simulink model "Projekt_simulink_v2"  (R2024b)
settings: Solver=VariableStepAuto  StartTime=0.0  StopTime=150  RelTol=1e-8
values from neighbouring files (symbols this model uses):
  A = zeros(12)    [pokus_simulink.m]
  B = zeros(12, 4)    [pokus_simulink.m]
  C = eye(12)    [pokus_simulink.m]
  D = zeros(12, 4)    [pokus_simulink.m]
  g = 9.81    [pokus_simulink.m]
  Mass = 1.3    [pokus_simulink.m]
libraries: slpidlib x3
settings Model: Creator=lucie  LastModifiedBy=lucie

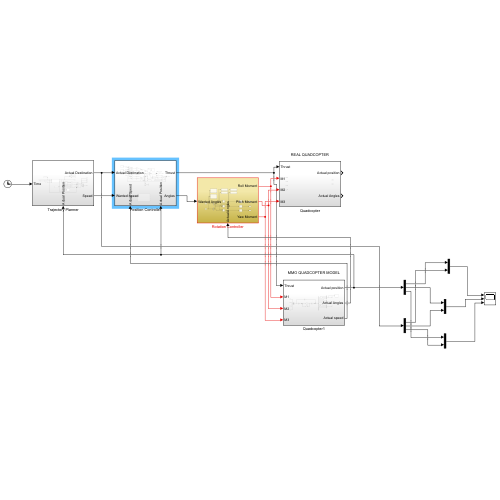
[thumbnail: Simulink's stored preview of the top-level diagram]
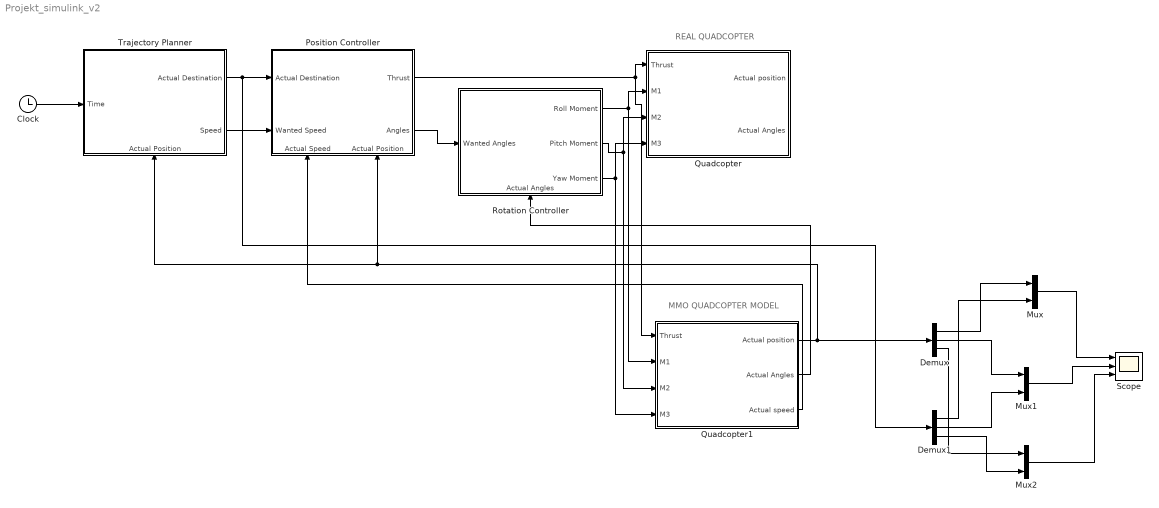
== system Projekt_simulink_v2 ==
  note: REAL QUADCOPTER
  note: MMO QUADCOPTER MODEL
  Clock : Clock
  Demux : Demux  Outputs=3
  Demux1 : Demux  Outputs=3
  Mux : Mux  Inputs=2
  Mux1 : Mux  Inputs=2
  Mux2 : Mux  Inputs=2
  Position Controller : Subsystem
      settings: PortSchema="{\"entries\":[{\"content\":{\"sides\":[{\"content\":{\"connectorIds\":[\"In1\",\"In2\"]},\"type\":\"ConnectorPlacement.EquallySpacedRectSide\",\"uuid\":\"80f29ff0-56da-481e-95f1-a9d4517a9ed9\"},{\"content\":{\"connectorIds\":[\"Out1\",\"Out2\"],\"side\":\"RIGHT\"},\"type\":\"ConnectorPlacement.EquallySpacedRectSide\",\"uuid\":\"630d0718-5a0f-420d-89e4-ff766e1306d8\"},{\"content\":{\"side\":\"TOP\"},\"type\":\"ConnectorPlacement.EquallySpacedRectSide\",\"uuid\":\"1f5a52b9-8732-4ff3-b402-4000d2af11bc\"},{\"content\":{\"connectorIds\":[\"In3\",\"In4\"],\"side\":\"BOTTOM\"},\"type\":\"ConnectorPlacement.EquallySpacedRectSide\",\"uuid\":\"db5f8e2a-d0de-4587-b83f-8eeb0fa2830b\"}]},\"type\":\"ConnectorPlacement.EquallySpacedConnector\",\"uuid\":\"97645df6-1a74-4cc0-aee4-69f235aa0ffb\"}],\"packageUris\":[\"http://schema.mathworks.com/mf0/Connector/R2020b\"],\"version\":\"1.0\"}"
  Quadcopter : Subsystem
  Quadcopter1 : Subsystem
  Rotation Controller : Subsystem
      settings: PortSchema="{\"entries\":[{\"content\":{\"sides\":[{\"content\":{\"connectorIds\":[\"In1\"]},\"type\":\"ConnectorPlacement.EquallySpacedRectSide\",\"uuid\":\"80f29ff0-56da-481e-95f1-a9d4517a9ed9\"},{\"content\":{\"connectorIds\":[\"Out1\",\"Out2\",\"Out3\"],\"side\":\"RIGHT\"},\"type\":\"ConnectorPlacement.EquallySpacedRectSide\",\"uuid\":\"630d0718-5a0f-420d-89e4-ff766e1306d8\"},{\"content\":{\"side\":\"TOP\"},\"type\":\"ConnectorPlacement.EquallySpacedRectSide\",\"uuid\":\"1f5a52b9-8732-4ff3-b402-4000d2af11bc\"},{\"content\":{\"connectorIds\":[\"In2\"],\"side\":\"BOTTOM\"},\"type\":\"ConnectorPlacement.EquallySpacedRectSide\",\"uuid\":\"db5f8e2a-d0de-4587-b83f-8eeb0fa2830b\"}]},\"type\":\"ConnectorPlacement.EquallySpacedConnector\",\"uuid\":\"97645df6-1a74-4cc0-aee4-69f235aa0ffb\"}],\"packageUris\":[\"http://schema.mathworks.com/mf0/Connector/R2020b\"],\"version\":\"1.0\"}"
  Scope : Scope  NumInputPorts=3
  Trajectory Planner : Subsystem
      settings: PortSchema="{\"entries\":[{\"content\":{\"sides\":[{\"content\":{\"connectorIds\":[\"In1\"]},\"type\":\"ConnectorPlacement.EquallySpacedRectSide\",\"uuid\":\"80f29ff0-56da-481e-95f1-a9d4517a9ed9\"},{\"content\":{\"connectorIds\":[\"Out1\",\"Out2\"],\"side\":\"RIGHT\"},\"type\":\"ConnectorPlacement.EquallySpacedRectSide\",\"uuid\":\"630d0718-5a0f-420d-89e4-ff766e1306d8\"},{\"content\":{\"side\":\"TOP\"},\"type\":\"ConnectorPlacement.EquallySpacedRectSide\",\"uuid\":\"1f5a52b9-8732-4ff3-b402-4000d2af11bc\"},{\"content\":{\"connectorIds\":[\"In2\"],\"side\":\"BOTTOM\"},\"type\":\"ConnectorPlacement.EquallySpacedRectSide\",\"uuid\":\"db5f8e2a-d0de-4587-b83f-8eeb0fa2830b\"}]},\"type\":\"ConnectorPlacement.EquallySpacedConnector\",\"uuid\":\"97645df6-1a74-4cc0-aee4-69f235aa0ffb\"}],\"packageUris\":[\"http://schema.mathworks.com/mf0/Connector/R2020b\"],\"version\":\"1.0\"}"
  wires:
  Trajectory Planner/1(Actual Destination) -> Demux1/1, Position Controller/1(Actual Destination)
  Trajectory Planner/2(Speed) -> Position Controller/2(Wanted Speed)
  Position Controller/2(Angles) -> Rotation Controller/1(Wanted Angles)
  Position Controller/1(Thrust) -> Quadcopter/1(Thrust), Quadcopter1/1(Thrust)
  Rotation Controller/1(Roll Moment) -> Quadcopter/2(M1), Quadcopter1/2(M1)
  Rotation Controller/2(Pitch Moment) -> Quadcopter1/3(M2), Quadcopter/3(M2)
  Rotation Controller/3(Yaw Moment) -> Quadcopter1/4(M3), Quadcopter/4(M3)
  Quadcopter1/2(Actual Angles) -> Rotation Controller/2(Actual Angles)
  Quadcopter1/3(Actual speed) -> Position Controller/3(Actual Speed)
  Clock/1 -> Trajectory Planner/1(Time)
  Quadcopter1/1(Actual position) -> Position Controller/4(Actual Position), Trajectory Planner/2(Actual Position), Demux/1
  Demux/1 -> Mux/1
  Demux1/1 -> Mux/2
  Demux/2 -> Mux1/1
  Demux1/2 -> Mux1/2
  Demux/3 -> Mux2/1
  Demux1/3 -> Mux2/2
  Mux/1 -> Scope/1
  Mux1/1 -> Scope/2
  Mux2/1 -> Scope/3

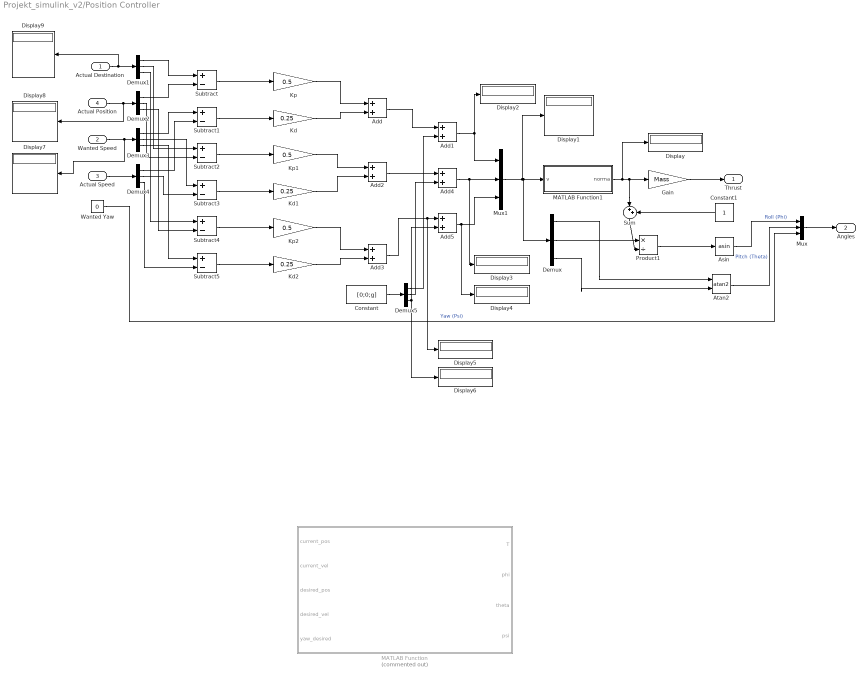
== system Projekt_simulink_v2/Position Controller ==
  Actual Destination : Inport
  Wanted Speed : Inport  Port=2
  Actual Speed : Inport  Port=3
  Actual Position : Inport  Port=4
  Add{,1..5} (6 alike) : Sum
  Asin : Trigonometry  Operator=asin
  Atan2 : Trigonometry  Operator=atan2
  Constant : Constant  Value=[0;0;g]
  Constant1 : Constant
  Demux{,1..5} (6 alike) : Demux  Outputs=3
  Display{,1..9} (10 alike) : Display
  Gain : Gain  Gain=Mass
  Kd : Gain  Gain=0.25
  Kd1 : Gain  Gain=0.25
  Kd2 : Gain  Gain=0.25
  Kp : Gain  Gain=0.5
  Kp1 : Gain  Gain=0.5
  Kp2 : Gain  Gain=0.5
  MATLAB Function : MATLAB Function  Commented=on  TreatAsAtomicUnit=on
  MATLAB Function1 : MATLAB Function  TreatAsAtomicUnit=on
  Mux : Mux  Inputs=3
  Mux1 : Mux  Inputs=3
  Product1 : Product  Inputs=*/
  Subtract{,1..5} (6 alike) : Sum  Inputs=+-
  Sum : Sum  Inputs=|++
  Wanted Yaw : Constant  Value=0
  Thrust : Outport
  Angles : Outport  Port=2
  wires:
  Mux/1 -> Angles/1
  Subtract/1 -> Kp/1
  Subtract1/1 -> Kd/1
  Kp/1 -> Add/1
  Kd/1 -> Add/2
  Gain/1 -> Thrust/1
  Actual Destination/1 -> Display9/1, Demux1/1
  Actual Position/1 -> Display8/1, Demux2/1
  Wanted Speed/1 -> Display7/1, Demux3/1
  Actual Speed/1 -> Demux4/1
  Demux1/1 -> Subtract/1
  Demux2/1 -> Subtract/2
  Demux3/1 -> Subtract1/1
  Demux4/1 -> Subtract1/2
  Kd1/1 -> Add2/2
  Subtract3/1 -> Kd1/1
  Kp1/1 -> Add2/1
  Kd2/1 -> Add3/2
  Subtract5/1 -> Kd2/1
  Kp2/1 -> Add3/1
  Subtract4/1 -> Kp2/1
  Subtract2/1 -> Kp1/1
  Demux1/2 -> Subtract2/1
  Demux2/2 -> Subtract2/2
  Demux3/2 -> Subtract3/1
  Demux4/2 -> Subtract3/2
  Demux1/3 -> Subtract4/1
  Demux2/3 -> Subtract4/2
  Demux3/3 -> Subtract5/1
  Demux4/3 -> Subtract5/2
  Constant/1 -> Demux5/1
  Add/1 -> Add1/1
  Demux5/1 -> Add1/2
  Demux5/2 -> Add4/2
  Demux5/3 -> Add5/2, Display6/1
  Add3/1 -> Display5/1, Add5/1
  Add2/1 -> Add4/1
  Add1/1 -> Display2/1, Mux1/1
  Add4/1 -> Display3/1, Mux1/2
  Add5/1 -> Display4/1, Mux1/3
  Mux1/1 -> Display1/1, Demux/1, MATLAB Function1/1(v)
  MATLAB Function1/1(norma) -> Display/1, Sum/1, Gain/1
  Demux/2 -> Product1/1
  Product1/1 -> Asin/1
  Asin/1 -> Mux/1  "Roll (Phi)"
  Demux/1 -> Atan2/1
  Demux/3 -> Atan2/2
  Atan2/1 -> Mux/2  "Pitch (Theta)"
  Wanted Yaw/1 -> Mux/3  "Yaw (Psi)"
  Constant1/1 -> Sum/2
  Sum/1 -> Product1/2

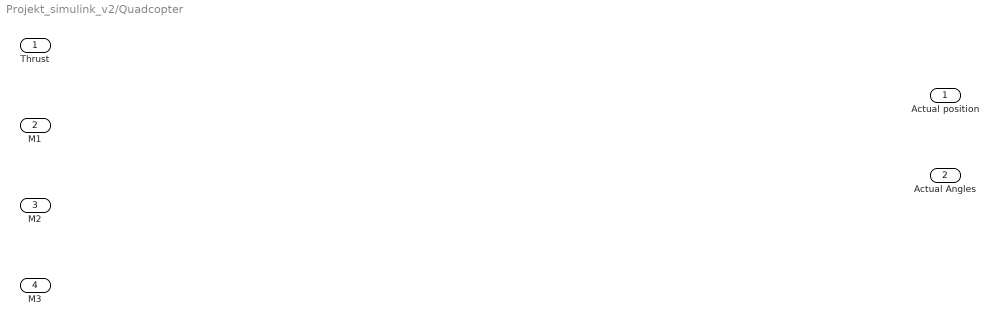
== system Projekt_simulink_v2/Quadcopter ==
  Thrust : Inport
  M1 : Inport  Port=2
  M2 : Inport  Port=3
  M3 : Inport  Port=4
  Actual position : Outport
  Actual Angles : Outport  Port=2

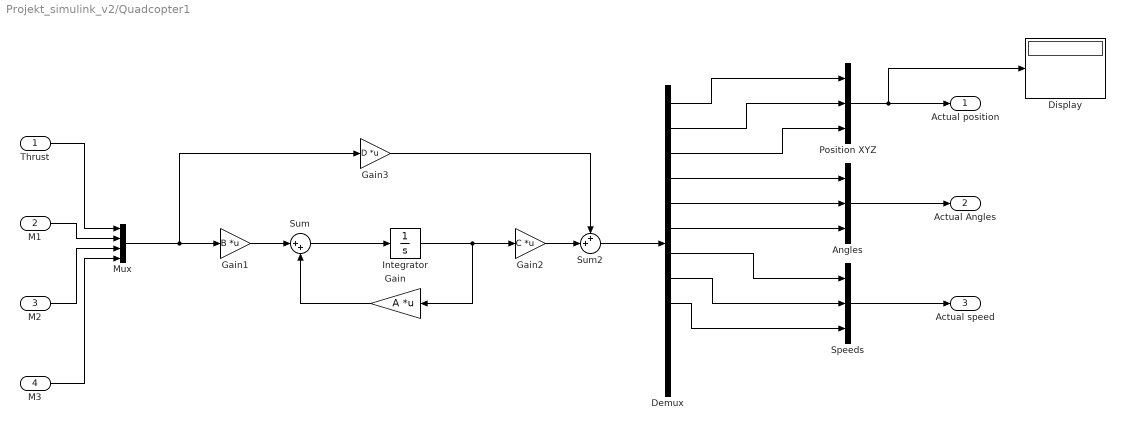
== system Projekt_simulink_v2/Quadcopter1 ==
  Thrust : Inport
  M1 : Inport  Port=2
  M2 : Inport  Port=3
  M3 : Inport  Port=4
  Angles : Mux  Inputs=3
  Demux : Demux  Outputs=12
  Display : Display
  Gain : Gain  Gain=A  Multiplication=Matrix(K*u)
  Gain1 : Gain  Gain=B  Multiplication=Matrix(K*u)
  Gain2 : Gain  Gain=C  Multiplication=Matrix(K*u)
  Gain3 : Gain  Gain=D  Multiplication=Matrix(K*u)
  Integrator : Integrator  InitialCondition=[0 0 -6 0 0 0 0 0 0 0 0 0]
  Mux : Mux
  Position XYZ : Mux  Inputs=3
  Speeds : Mux  Inputs=3
  Sum : Sum  Inputs=|++
  Sum2 : Sum  Inputs=++|
  Actual position : Outport
  Actual Angles : Outport  Port=2
  Actual speed : Outport  Port=3
  wires:
  Gain/1 -> Sum/2
  Gain1/1 -> Sum/1
  Sum/1 -> Integrator/1
  Integrator/1 -> Gain/1, Gain2/1
  Gain2/1 -> Sum2/2
  Gain3/1 -> Sum2/1
  Thrust/1 -> Mux/1
  M1/1 -> Mux/2
  M2/1 -> Mux/3
  M3/1 -> Mux/4
  Mux/1 -> Gain3/1, Gain1/1
  Sum2/1 -> Demux/1
  Demux/1 -> Position XYZ/1
  Demux/3 -> Position XYZ/3
  Demux/2 -> Position XYZ/2
  Position XYZ/1 -> Display/1, Actual position/1
  Demux/4 -> Angles/1
  Demux/5 -> Angles/2
  Demux/6 -> Angles/3
  Angles/1 -> Actual Angles/1
  Demux/7 -> Speeds/1
  Demux/8 -> Speeds/2
  Demux/9 -> Speeds/3
  Speeds/1 -> Actual speed/1

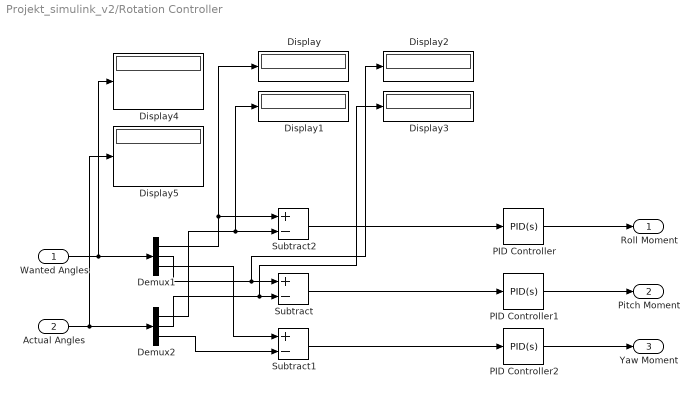
== system Projekt_simulink_v2/Rotation Controller ==
  Wanted Angles : Inport
  Actual Angles : Inport  Port=2
  Demux1 : Demux  Outputs=3
  Demux2 : Demux  Outputs=3
  Display{,1..5} (6 alike) : Display
  PID Controller : slpidlib/PID Controller  Controller=PID  Form=Parallel  TimeDomain=Continuous-time  UseExternalTs=off  SampleTime=-1  IntegratorMethod=Forward Euler  FilterMethod=Forward Euler  ControllerParametersSource=internal  P=0.5  I=0.1  UseKiTs=off  D=0.05  UseExternalDerivativeSource=off  N=100  UseFilter=on  TunerSelectOption=Transfer Function Based (PID Tuner App)  InitialConditionSource=internal  InitialConditionForIntegrator=0  InitialConditionForFilter=0  DifferentiatorICPrevScaledInput=0  ExternalReset=none  TrackingMode=off  Kt=1  LimitOutput=off  SatLimitsSource=internal  UpperSaturationLimit=inf  LowerSaturationLimit=-inf  LinearizeAsGain=on  AntiWindupMode=none  Kb=1  LimitIntegrator=off  UpperIntegratorSaturationLimit=inf  LowerIntegratorSaturationLimit=-inf  POutMin=[]  POutMax=[]  IOutMin=[]  IOutMax=[]  DOutMin=[]  DOutMax=[]  NOutMin=[]  NOutMax=[]  SumOutMin=[]  SumOutMax=[]  SaturationOutMin=[]  SaturationOutMax=[]  PParamMin=[]  PParamMax=[]  IParamMin=[]  IParamMax=[]  DParamMin=[]  DParamMax=[]  NParamMin=[]  NParamMax=[]  KbParamMin=[]  KbParamMax=[]  KtParamMin=[]  KtParamMax=[]  KbOutMin=[]  KbOutMax=[]  KtOutMin=[]  KtOutMax=[]  IntegratorOutMin=[]  IntegratorOutMax=[]  FilterOutMin=[]  FilterOutMax=[]  SumI1OutMin=[]  SumI1OutMax=[]  SumI2OutMin=[]  SumI2OutMax=[]  SumI3OutMin=[]  SumI3OutMax=[]  SumI4OutMin=[]  SumI4OutMax=[]  SumDOutMin=[]  SumDOutMax=[]  DifferentiatorOutMin=[]  DifferentiatorOutMax=[]  FilterDiffOutCoefMin=[]  FilterDiffOutCoefMax=[]  ReciprocalOutMin=[]  ReciprocalOutMax=[]  SumDenOutMin=[]  SumDenOutMax=[]  SumNumOutMin=[]  SumNumOutMax=[]  DivideOutMin=[]  DivideOutMax=[]  UdiffTsProdOutMin=[]  UdiffTsProdOutMax=[]  NTsProdOutMin=[]  NTsProdOutMax=[]  UintegralTsProdOutMin=[]  UintegralTsProdOutMax=[]  UngainTsProdOutMin=[]  UngainTsProdOutMax=[]  ClampingZeroOutDataTypeStr=Inherit: Inherit via back propagation  ClampingZeroOutMin=[]  ClampingZeroOutMax=[]  FilterDenConstantOutDataTypeStr=Inherit: Inherit via back propagation  FilterDenConstantOutMin=[]  FilterDenConstantOutMax=[]  PCopyOutDataTypeStr=Inherit: Inherit via back propagation  PCopyOutMin=[]  PCopyOutMax=[]  NCopyOutDataTypeStr=Inherit: Inherit via back propagation  NCopyOutMin=[]  NCopyOutMax=[]  IntegratorContinuousStateAttributes=''  IntegratorStateMustResolveToSignalObject=off  IntegratorRTWStateStorageClass=Auto  FilterContinuousStateAttributes=''  FilterStateMustResolveToSignalObject=off  FilterRTWStateStorageClass=Auto  ParallelPVariant=InternalParameters  IdealPVariant=Disabled  IVariant=InternalParameters  DVariant=InternalParameters  IntegratorVariant=Continuous  SatVariant=Disabled  AWVariant=Passthrough  PCopyVariant=Disabled  TRVariant=Disabled  FdbkBlocksVariant=Forward  IdealPFdbkVariant=Disabled  SatFdbkVariant=Disabled  DerivativeFilterVariant=ContFilter  NVariant=InternalParameters  NCopyVariant=Disabled  FilterICVariant=InternalICsFilter  IntegratorICVariant=InternalICs  ExternalResetVariant=Disabled  TRSumVariant=Passthrough  SumFdbkVariant=Disabled  SumVariant=Sum_PID  TsampFilterVariant=InternalTs  TsampNgainVariant=Passthrough  TsampIntegralVariant=Disabled_SignalSpec  ExternalSaturationOutDataTypeStr=Inherit: Same as second input  DerivativeSourceVariant=ErrorSignal  PreIntVariant=InternalPreInt
  PID Controller1 : slpidlib/PID Controller  Controller=PID  Form=Parallel  TimeDomain=Continuous-time  UseExternalTs=off  SampleTime=-1  IntegratorMethod=Forward Euler  FilterMethod=Forward Euler  ControllerParametersSource=internal  P=0.5  I=0.1  UseKiTs=off  D=0.05  UseExternalDerivativeSource=off  N=100  UseFilter=on  TunerSelectOption=Transfer Function Based (PID Tuner App)  InitialConditionSource=internal  InitialConditionForIntegrator=0  InitialConditionForFilter=0  DifferentiatorICPrevScaledInput=0  ExternalReset=none  TrackingMode=off  Kt=1  LimitOutput=off  SatLimitsSource=internal  UpperSaturationLimit=inf  LowerSaturationLimit=-inf  LinearizeAsGain=on  AntiWindupMode=none  Kb=1  LimitIntegrator=off  UpperIntegratorSaturationLimit=inf  LowerIntegratorSaturationLimit=-inf  POutMin=[]  POutMax=[]  IOutMin=[]  IOutMax=[]  DOutMin=[]  DOutMax=[]  NOutMin=[]  NOutMax=[]  SumOutMin=[]  SumOutMax=[]  SaturationOutMin=[]  SaturationOutMax=[]  PParamMin=[]  PParamMax=[]  IParamMin=[]  IParamMax=[]  DParamMin=[]  DParamMax=[]  NParamMin=[]  NParamMax=[]  KbParamMin=[]  KbParamMax=[]  KtParamMin=[]  KtParamMax=[]  KbOutMin=[]  KbOutMax=[]  KtOutMin=[]  KtOutMax=[]  IntegratorOutMin=[]  IntegratorOutMax=[]  FilterOutMin=[]  FilterOutMax=[]  SumI1OutMin=[]  SumI1OutMax=[]  SumI2OutMin=[]  SumI2OutMax=[]  SumI3OutMin=[]  SumI3OutMax=[]  SumI4OutMin=[]  SumI4OutMax=[]  SumDOutMin=[]  SumDOutMax=[]  DifferentiatorOutMin=[]  DifferentiatorOutMax=[]  FilterDiffOutCoefMin=[]  FilterDiffOutCoefMax=[]  ReciprocalOutMin=[]  ReciprocalOutMax=[]  SumDenOutMin=[]  SumDenOutMax=[]  SumNumOutMin=[]  SumNumOutMax=[]  DivideOutMin=[]  DivideOutMax=[]  UdiffTsProdOutMin=[]  UdiffTsProdOutMax=[]  NTsProdOutMin=[]  NTsProdOutMax=[]  UintegralTsProdOutMin=[]  UintegralTsProdOutMax=[]  UngainTsProdOutMin=[]  UngainTsProdOutMax=[]  ClampingZeroOutDataTypeStr=Inherit: Inherit via back propagation  ClampingZeroOutMin=[]  ClampingZeroOutMax=[]  FilterDenConstantOutDataTypeStr=Inherit: Inherit via back propagation  FilterDenConstantOutMin=[]  FilterDenConstantOutMax=[]  PCopyOutDataTypeStr=Inherit: Inherit via back propagation  PCopyOutMin=[]  PCopyOutMax=[]  NCopyOutDataTypeStr=Inherit: Inherit via back propagation  NCopyOutMin=[]  NCopyOutMax=[]  IntegratorContinuousStateAttributes=''  IntegratorStateMustResolveToSignalObject=off  IntegratorRTWStateStorageClass=Auto  FilterContinuousStateAttributes=''  FilterStateMustResolveToSignalObject=off  FilterRTWStateStorageClass=Auto  ParallelPVariant=InternalParameters  IdealPVariant=Disabled  IVariant=InternalParameters  DVariant=InternalParameters  IntegratorVariant=Continuous  SatVariant=Disabled  AWVariant=Passthrough  PCopyVariant=Disabled  TRVariant=Disabled  FdbkBlocksVariant=Forward  IdealPFdbkVariant=Disabled  SatFdbkVariant=Disabled  DerivativeFilterVariant=ContFilter  NVariant=InternalParameters  NCopyVariant=Disabled  FilterICVariant=InternalICsFilter  IntegratorICVariant=InternalICs  ExternalResetVariant=Disabled  TRSumVariant=Passthrough  SumFdbkVariant=Disabled  SumVariant=Sum_PID  TsampFilterVariant=InternalTs  TsampNgainVariant=Passthrough  TsampIntegralVariant=Disabled_SignalSpec  ExternalSaturationOutDataTypeStr=Inherit: Same as second input  DerivativeSourceVariant=ErrorSignal  PreIntVariant=InternalPreInt
  PID Controller2 : slpidlib/PID Controller  Controller=PID  Form=Parallel  TimeDomain=Continuous-time  UseExternalTs=off  SampleTime=-1  IntegratorMethod=Forward Euler  FilterMethod=Forward Euler  ControllerParametersSource=internal  P=0.3  I=0.05  UseKiTs=off  D=0.02  UseExternalDerivativeSource=off  N=100  UseFilter=on  TunerSelectOption=Transfer Function Based (PID Tuner App)  InitialConditionSource=internal  InitialConditionForIntegrator=0  InitialConditionForFilter=0  DifferentiatorICPrevScaledInput=0  ExternalReset=none  TrackingMode=off  Kt=1  LimitOutput=off  SatLimitsSource=internal  UpperSaturationLimit=inf  LowerSaturationLimit=-inf  LinearizeAsGain=on  AntiWindupMode=none  Kb=1  LimitIntegrator=off  UpperIntegratorSaturationLimit=inf  LowerIntegratorSaturationLimit=-inf  POutMin=[]  POutMax=[]  IOutMin=[]  IOutMax=[]  DOutMin=[]  DOutMax=[]  NOutMin=[]  NOutMax=[]  SumOutMin=[]  SumOutMax=[]  SaturationOutMin=[]  SaturationOutMax=[]  PParamMin=[]  PParamMax=[]  IParamMin=[]  IParamMax=[]  DParamMin=[]  DParamMax=[]  NParamMin=[]  NParamMax=[]  KbParamMin=[]  KbParamMax=[]  KtParamMin=[]  KtParamMax=[]  KbOutMin=[]  KbOutMax=[]  KtOutMin=[]  KtOutMax=[]  IntegratorOutMin=[]  IntegratorOutMax=[]  FilterOutMin=[]  FilterOutMax=[]  SumI1OutMin=[]  SumI1OutMax=[]  SumI2OutMin=[]  SumI2OutMax=[]  SumI3OutMin=[]  SumI3OutMax=[]  SumI4OutMin=[]  SumI4OutMax=[]  SumDOutMin=[]  SumDOutMax=[]  DifferentiatorOutMin=[]  DifferentiatorOutMax=[]  FilterDiffOutCoefMin=[]  FilterDiffOutCoefMax=[]  ReciprocalOutMin=[]  ReciprocalOutMax=[]  SumDenOutMin=[]  SumDenOutMax=[]  SumNumOutMin=[]  SumNumOutMax=[]  DivideOutMin=[]  DivideOutMax=[]  UdiffTsProdOutMin=[]  UdiffTsProdOutMax=[]  NTsProdOutMin=[]  NTsProdOutMax=[]  UintegralTsProdOutMin=[]  UintegralTsProdOutMax=[]  UngainTsProdOutMin=[]  UngainTsProdOutMax=[]  ClampingZeroOutDataTypeStr=Inherit: Inherit via back propagation  ClampingZeroOutMin=[]  ClampingZeroOutMax=[]  FilterDenConstantOutDataTypeStr=Inherit: Inherit via back propagation  FilterDenConstantOutMin=[]  FilterDenConstantOutMax=[]  PCopyOutDataTypeStr=Inherit: Inherit via back propagation  PCopyOutMin=[]  PCopyOutMax=[]  NCopyOutDataTypeStr=Inherit: Inherit via back propagation  NCopyOutMin=[]  NCopyOutMax=[]  IntegratorContinuousStateAttributes=''  IntegratorStateMustResolveToSignalObject=off  IntegratorRTWStateStorageClass=Auto  FilterContinuousStateAttributes=''  FilterStateMustResolveToSignalObject=off  FilterRTWStateStorageClass=Auto  ParallelPVariant=InternalParameters  IdealPVariant=Disabled  IVariant=InternalParameters  DVariant=InternalParameters  IntegratorVariant=Continuous  SatVariant=Disabled  AWVariant=Passthrough  PCopyVariant=Disabled  TRVariant=Disabled  FdbkBlocksVariant=Forward  IdealPFdbkVariant=Disabled  SatFdbkVariant=Disabled  DerivativeFilterVariant=ContFilter  NVariant=InternalParameters  NCopyVariant=Disabled  FilterICVariant=InternalICsFilter  IntegratorICVariant=InternalICs  ExternalResetVariant=Disabled  TRSumVariant=Passthrough  SumFdbkVariant=Disabled  SumVariant=Sum_PID  TsampFilterVariant=InternalTs  TsampNgainVariant=Passthrough  TsampIntegralVariant=Disabled_SignalSpec  ExternalSaturationOutDataTypeStr=Inherit: Same as second input  DerivativeSourceVariant=ErrorSignal  PreIntVariant=InternalPreInt
  Subtract : Sum  Inputs=+-
  Subtract1 : Sum  Inputs=+-
  Subtract2 : Sum  Inputs=+-
  Roll Moment : Outport
  Pitch Moment : Outport  Port=2
  Yaw Moment : Outport  Port=3
  wires:
  Wanted Angles/1 -> Display4/1, Demux1/1
  Subtract1/1 -> PID Controller2/1
  Subtract/1 -> PID Controller1/1
  Subtract2/1 -> PID Controller/1
  PID Controller/1 -> Roll Moment/1
  PID Controller1/1 -> Pitch Moment/1
  PID Controller2/1 -> Yaw Moment/1
  Actual Angles/1 -> Demux2/1, Display5/1
  Demux1/1 -> Display/1, Subtract2/1
  Demux2/1 -> Display1/1, Subtract2/2
  Demux1/2 -> Display2/1, Subtract/1
  Demux2/2 -> Display3/1, Subtract/2
  Demux1/3 -> Subtract1/1
  Demux2/3 -> Subtract1/2

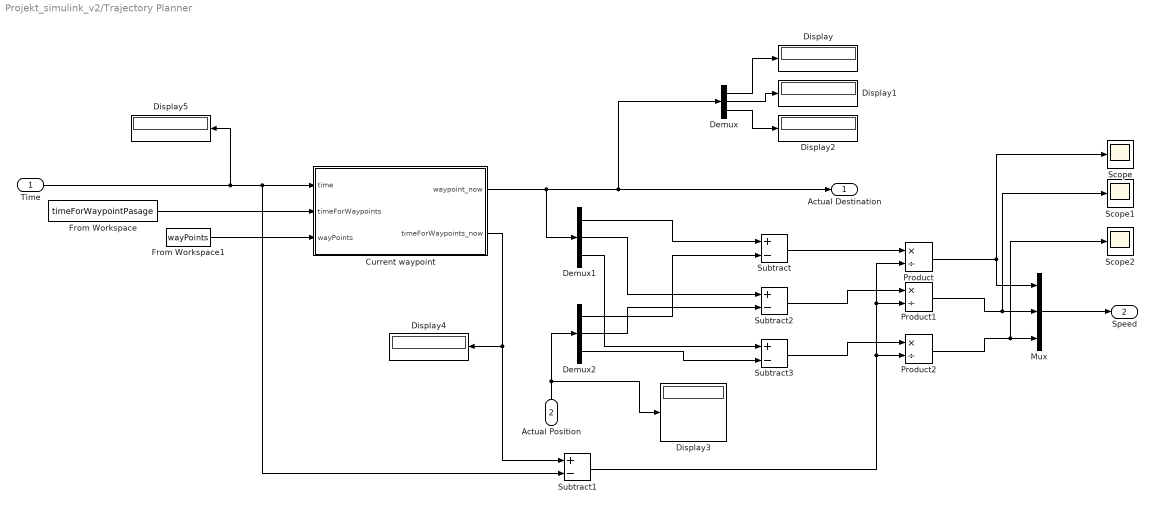
== system Projekt_simulink_v2/Trajectory Planner ==
  Time : Inport
  Actual Position : Inport  Port=2
  Current waypoint : MATLAB Function  TreatAsAtomicUnit=on
  Demux : Demux  Outputs=3
  Demux1 : Demux  Outputs=3
  Demux2 : Demux  Outputs=3
  Display{,1..5} (6 alike) : Display
  From Workspace : FromWorkspace  VariableName=timeForWaypointPasage
  From Workspace1 : FromWorkspace  VariableName=wayPoints
  Mux : Mux  Inputs=3
  Product : Product  Inputs=*/
  Product1 : Product  Inputs=*/
  Product2 : Product  Inputs=*/
  Scope : Scope
  Scope1 : Scope
  Scope2 : Scope
  Subtract{,1..3} (4 alike) : Sum  Inputs=+-
  Actual Destination : Outport
  Speed : Outport  Port=2
  wires:
  Time/1 -> Display5/1, Subtract1/2, Current waypoint/1(time)
  From Workspace/1 -> Current waypoint/2(timeForWaypoints)
  From Workspace1/1 -> Current waypoint/3(wayPoints)
  Current waypoint/1(waypoint_now) -> Demux1/1, Demux/1, Actual Destination/1
  Current waypoint/2(timeForWaypoints_now) -> Display4/1, Subtract1/1
  Product/1 -> Mux/1, Scope/1
  Demux/1 -> Display/1
  Demux/2 -> Display1/1
  Demux/3 -> Display2/1
  Actual Position/1 -> Demux2/1, Display3/1
  Demux1/1 -> Subtract/1
  Demux2/1 -> Subtract/2
  Demux1/2 -> Subtract2/1
  Demux2/2 -> Subtract2/2
  Demux1/3 -> Subtract3/1
  Demux2/3 -> Subtract3/2
  Subtract/1 -> Product/1
  Subtract2/1 -> Product1/1
  Subtract3/1 -> Product2/1
  Subtract1/1 -> Product1/2, Product/2, Product2/2
  Product1/1 -> Scope1/1, Mux/2
  Product2/1 -> Scope2/1, Mux/3
  Mux/1 -> Speed/1

== matlab function Projekt_simulink_v2/Position Controller/MATLAB Function ==
  data: current_pos input; T output; current_vel input; desired_pos input; desired_vel input; phi output; theta output; psi output; yaw_desired input
function [T, phi, theta, psi] = calculateThrustAndAngles(current_pos, current_vel, desired_pos, desired_vel, yaw_desired)
    
    g = 9.81;
    Kp = 0.5;
    Kd = 0.25;
    mass = 1.3;

    % Chyba polohy a rychlosti
    e_pos = desired_pos - current_pos;
    e_vel = desired_vel - current_vel;

    % Požadované zrychlení
    a_desired = Kp * e_pos + Kd * e_vel;

    % Celkové zrychlení včetně gravitace
    a_total = a_desired + [0; 0; g];

    % Tah (T)
    T = mass * norm(a_total);

    % Úhly natočení (phi, theta, psi)
    phi = asin(a_total(2) / norm(a_total));    % Roll
    theta = atan2(a_total(1), a_total(3));     % Pitch
    psi = yaw_desired;                         % Yaw je přímo požadovaný úhel
end

== matlab function Projekt_simulink_v2/Trajectory Planner/Current waypoint ==
  data: time input; waypoint_now output; timeForWaypoints input; wayPoints input; timeForWaypoints_now output
function [waypoint_now,timeForWaypoints_now]= fcn(time, timeForWaypoints, wayPoints)
    
    timeForWaypoints = [100,200,300,400,500]; % [s]

    % Waypoints - these points must be flown by quadcopter
    wayPoints = [0 0 -6;        % [X, Y, Z] - waypoint in [m]
             1 1 -10;
             1 2 -4;
             2 2 -5;
             3 1 -6];
    
    % Počet waypointů
    numWaypoints = size(wayPoints, 1);

    % Defaultní waypoint, pokud čas simulace přesáhne všechny časy
    waypoint_now = wayPoints(end, :);
    timeForWaypoints_now = timeForWaypoints(end);

    % Najdeme odpovídající waypoint podle času
    for i = 1:numWaypoints
        if time <= timeForWaypoints(i)
            waypoint_now = wayPoints(i, :);
            timeForWaypoints_now = timeForWaypoints(i);
            return;
        end
    end
    
end

== matlab function Projekt_simulink_v2/Position Controller/MATLAB Function1 ==
  data: v input; norma output
function norma = vector_norm(v)
    norma = norm(v);
end
